simulink model "weekproblem9"  (R2020b)
settings: Solver=VariableStepAuto  StartTime=0.0  StopTime=10  RelTol=1e-3
values from neighbouring files (symbols this model uses):
  b = 0.1    [parameters.m]
  J = 0.01    [parameters.m]
  L = 0.5    [parameters.m]
  R = 1    [parameters.m]
settings Model: Creator=Puru Gawande  LastModifiedBy=Puru Gawande

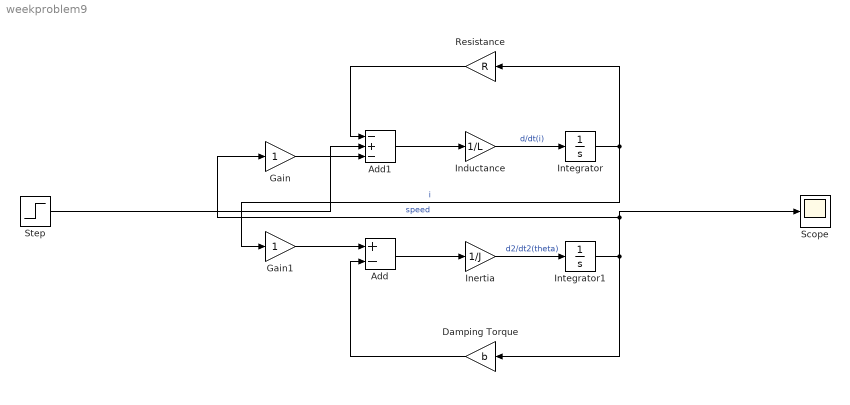
== system weekproblem9 ==
  Add : Sum  Inputs=+-
  Add1 : Sum  Inputs=-+-
  Damping Torque : Gain  Gain=b
  Gain : Gain
  Gain1 : Gain
  Inductance : Gain  Gain=1/L
  Inertia : Gain  Gain=1/J
  Integrator : Integrator
  Integrator1 : Integrator
  Resistance : Gain  Gain=R
  Scope : Scope
  Step : Step  SampleTime=0
  wires:
  Damping Torque/1 -> Add/2
  Inertia/1 -> Integrator1/1  "d2/dt2(theta)"
  Gain/1 -> Add1/3
  Integrator1/1 -> Scope/1, Gain/1, Damping Torque/1  "speed"
  Gain1/1 -> Add/1
  Step/1 -> Add1/2
  Integrator/1 -> Gain1/1, Resistance/1  "i"
  Resistance/1 -> Add1/1
  Add/1 -> Inertia/1
  Add1/1 -> Inductance/1
  Inductance/1 -> Integrator/1  "d/dt(i)"
